simulink model "BalanceTest_MDL"  (R2016b)
settings: Solver=FixedStepAuto  StartTime=0.0  StopTime=inf  FixedStep=0.02  RelTol=1e-3
values from neighbouring files (symbols this model uses):
  alpha_comp = 0.98    [ModelSetup.m]
  K_phi = 2.42    [ModelSetup.m]
  K_u_K = 0.3    [ModelSetup.m]
  K_u_R = 0.0008    [ModelSetup.m]
  phi_max = degtorad(10)    [ModelSetup.m]
  r_S1 = 0.14    [ModelSetup.m]
  r_S2 = 0.061    [ModelSetup.m]
  Ta = 0.02    [ModelSetup.m]
undefined symbols (not defined in the file or in its folder): adc_poly, w1_poly, w2_poly, x1_poly, x2_poly, y1_poly, y2_poly
libraries: MSCubeLibrary x3, simulink x1
settings Model: SimulationMode=external  Creator=ich  LastModifiedBy=ich
settings OptimizationCC: MaxStackSize=64
settings DebuggingCC: ParameterTunabilityLossMsg=error
settings HardwareCC: ProdBitPerPointer=32  ProdBitPerSizeT=32  ProdBitPerPtrDiffT=32  ProdLargestAtomicInteger=Long  ProdLargestAtomicFloat=Double  ProdWordSize=32  ProdHWDeviceType=ARM Compatible->ARM Cortex
settings RTWCC: SystemTargetFile=ert.tlc  HardwareBoard=MSCubeBBB  TLCOptions="-aInlineSetEventsForThisBaseRateFcn=TLC_FALSE -aSuppressMultiTaskScheduler=TLC_FALSE  -aRateBasedStepFcn=0"  TemplateMakefile=ert_default_tmf  Description=Embedded Coder  GenerateReport=on  Toolchain=Linaro Toolchain v4.8  IncludeHyperlinkInReport=on  LaunchReport=on  GenerateTraceInfo=on  GenerateTraceReport=on  GenerateTraceReportSl=on  GenerateTraceReportSf=on  GenerateTraceReportEml=on
settings CodeAppCC: ForceParamTrailComments=on  IgnoreCustomStorageClasses=off  OperatorAnnotations=on  SimulinkDataObjDesc=on  SFDataObjDesc=on  MATLABFcnDesc=on  InsertBlockDesc=on  MATLABSourceComments=on

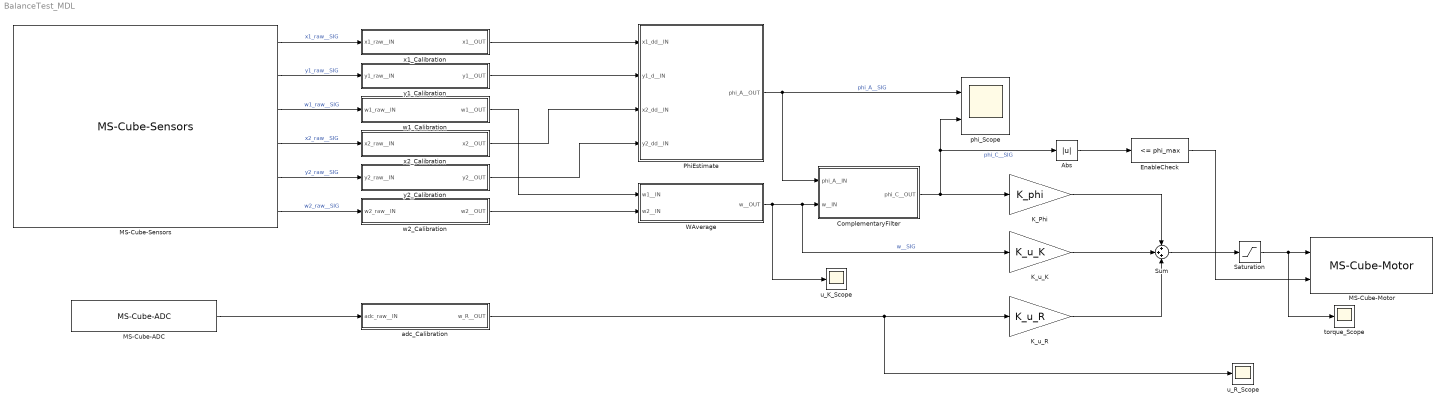
== system BalanceTest_MDL ==
  Abs : Abs
  ComplementaryFilter : Subsystem
  EnableCheck : simulink/Logic and Bit Operations/Compare To Constant  relop=<=  const=phi_max  OutDataTypeStr=boolean
  K_Phi : Gain  Gain=K_phi
  K_u_K : Gain  Gain=K_u_K
  K_u_R : Gain  Gain=K_u_R
  MS-Cube-ADC : MSCubeLibrary/MS-Cube-ADC
  MS-Cube-Motor : MSCubeLibrary/MS-Cube-Motor
  MS-Cube-Sensors : MSCubeLibrary/MS-Cube-Sensors
  PhiEstimate : Subsystem
  Saturation : Saturate  UpperLimit=0.11  LowerLimit=-0.11  OutDataTypeStr=single
  Sum : Sum  Inputs=+++  OutDataTypeStr=single
  WAverage : Subsystem
  adc_Calibration : Subsystem
  phi_Scope : Scope  NumInputPorts=2
  torque_Scope : Scope
  u_K_Scope : Scope
  u_R_Scope : Scope
  w1_Calibration : Subsystem
  w2_Calibration : Subsystem
  x1_Calibration : Subsystem
  x2_Calibration : Subsystem
  y1_Calibration : Subsystem
  y2_Calibration : Subsystem
  wires:
  MS-Cube-Sensors/1 -> x1_Calibration/1(x1_raw__IN)  "x1_raw__SIG"
  MS-Cube-Sensors/2 -> y1_Calibration/1(y1_raw__IN)  "y1_raw__SIG"
  MS-Cube-Sensors/3 -> w1_Calibration/1(w1_raw__IN)  "w1_raw__SIG"
  MS-Cube-Sensors/4 -> x2_Calibration/1(x2_raw__IN)  "x2_raw__SIG"
  MS-Cube-Sensors/5 -> y2_Calibration/1(y2_raw__IN)  "y2_raw__SIG"
  MS-Cube-Sensors/6 -> w2_Calibration/1(w2_raw__IN)  "w2_raw__SIG"
  x1_Calibration/1(x1__OUT) -> PhiEstimate/1(x1_dd__IN)
  y1_Calibration/1(y1__OUT) -> PhiEstimate/2(y1_d__IN)
  x2_Calibration/1(x2__OUT) -> PhiEstimate/3(x2_dd__IN)
  y2_Calibration/1(y2__OUT) -> PhiEstimate/4(y2_dd__IN)
  w2_Calibration/1(w2__OUT) -> WAverage/2(w2__IN)
  w1_Calibration/1(w1__OUT) -> WAverage/1(w1__IN)
  PhiEstimate/1(phi_A__OUT) -> ComplementaryFilter/1(phi_A__IN), phi_Scope/1  "phi_A__SIG"
  WAverage/1(w__OUT) -> u_K_Scope/1, K_u_K/1, ComplementaryFilter/2(w__IN)  "w__SIG"
  ComplementaryFilter/1(phi_C__OUT) -> K_Phi/1, phi_Scope/2, Abs/1  "phi_C__SIG"
  MS-Cube-ADC/1 -> adc_Calibration/1(adc_raw__IN)
  K_u_K/1 -> Sum/2
  K_Phi/1 -> Sum/1
  K_u_R/1 -> Sum/3
  adc_Calibration/1(w_R__OUT) -> u_R_Scope/1, K_u_R/1
  Sum/1 -> Saturation/1
  Abs/1 -> EnableCheck/1
  EnableCheck/1 -> MS-Cube-Motor/2
  Saturation/1 -> torque_Scope/1, MS-Cube-Motor/1

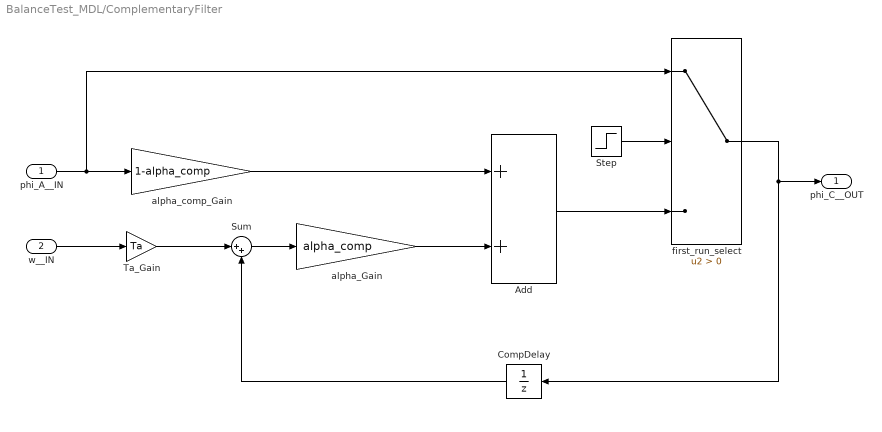
== system BalanceTest_MDL/ComplementaryFilter ==
  phi_A__IN : Inport
  w__IN : Inport  Port=2
  Add : Sum
  CompDelay : UnitDelay  SampleTime=Ta
  Step : Step  Time=Ta  Before=1  After=0  SampleTime=Ta
  Sum : Sum  Inputs=|++
  Ta_Gain : Gain  Gain=Ta
  alpha_Gain : Gain  Gain=alpha_comp
  alpha_comp_Gain : Gain  Gain=1-alpha_comp
  first_run_select : Switch  Criteria=u2 > Threshold
  phi_C__OUT : Outport
  wires:
  w__IN/1 -> Ta_Gain/1
  Ta_Gain/1 -> Sum/1
  Sum/1 -> alpha_Gain/1
  phi_A__IN/1 -> first_run_select/1, alpha_comp_Gain/1
  alpha_comp_Gain/1 -> Add/1
  alpha_Gain/1 -> Add/2
  Add/1 -> first_run_select/3
  first_run_select/1 -> CompDelay/1, phi_C__OUT/1
  CompDelay/1 -> Sum/2
  Step/1 -> first_run_select/2

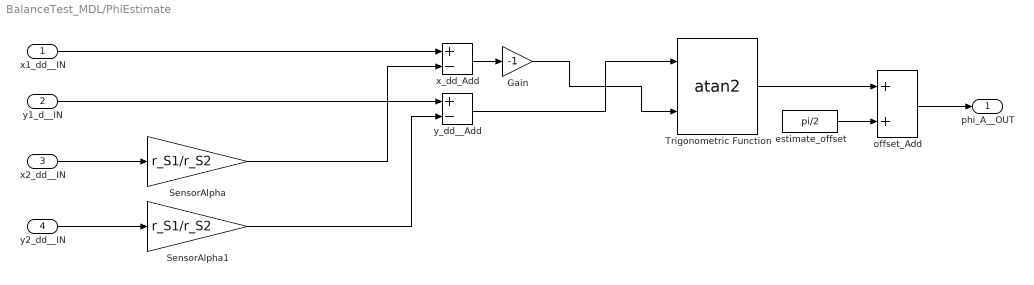
== system BalanceTest_MDL/PhiEstimate ==
  x1_dd__IN : Inport
  y1_d__IN : Inport  Port=2
  x2_dd__IN : Inport  Port=3
  y2_dd__IN : Inport  Port=4
  Gain : Gain  Gain=-1
  SensorAlpha : Gain  Gain=r_S1/r_S2
  SensorAlpha1 : Gain  Gain=r_S1/r_S2
  Trigonometric Function : Trigonometry  Operator=atan2
  estimate_offset : Constant  Value=pi/2
  offset_Add : Sum
  x_dd_Add : Sum  Inputs=+-
  y_dd__Add : Sum  Inputs=+-
  phi_A__OUT : Outport
  wires:
  x2_dd__IN/1 -> SensorAlpha/1
  y2_dd__IN/1 -> SensorAlpha1/1
  x1_dd__IN/1 -> x_dd_Add/1
  SensorAlpha/1 -> x_dd_Add/2
  y1_d__IN/1 -> y_dd__Add/1
  SensorAlpha1/1 -> y_dd__Add/2
  x_dd_Add/1 -> Gain/1
  y_dd__Add/1 -> Trigonometric Function/1
  Gain/1 -> Trigonometric Function/2
  Trigonometric Function/1 -> offset_Add/1
  estimate_offset/1 -> offset_Add/2
  offset_Add/1 -> phi_A__OUT/1

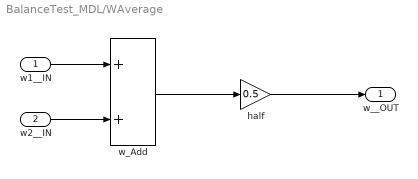
== system BalanceTest_MDL/WAverage ==
  w1__IN : Inport
  w2__IN : Inport  Port=2
  half : Gain  Gain=0.5
  w_Add : Sum
  w__OUT : Outport
  wires:
  w2__IN/1 -> w_Add/2
  w1__IN/1 -> w_Add/1
  w_Add/1 -> half/1
  half/1 -> w__OUT/1

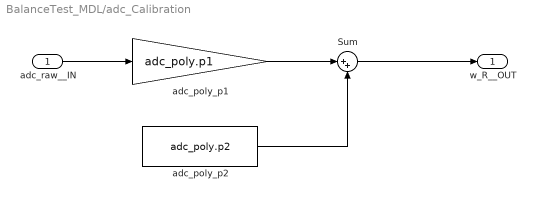
== system BalanceTest_MDL/adc_Calibration ==
  adc_raw__IN : Inport
  Sum : Sum  Inputs=|++
  adc_poly_p1 : Gain  Gain=adc_poly.p1
  adc_poly_p2 : Constant  Value=adc_poly.p2
  w_R__OUT : Outport
  wires:
  Sum/1 -> w_R__OUT/1
  adc_poly_p2/1 -> Sum/2
  adc_poly_p1/1 -> Sum/1
  adc_raw__IN/1 -> adc_poly_p1/1

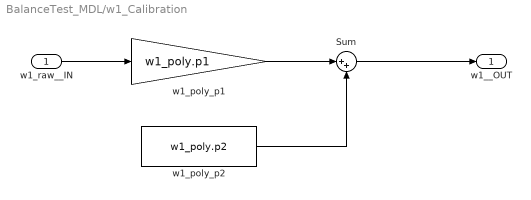
== system BalanceTest_MDL/w1_Calibration ==
  w1_raw__IN : Inport
  Sum : Sum  Inputs=|++
  w1_poly_p1 : Gain  Gain=w1_poly.p1
  w1_poly_p2 : Constant  Value=w1_poly.p2
  w1__OUT : Outport
  wires:
  Sum/1 -> w1__OUT/1
  w1_poly_p2/1 -> Sum/2
  w1_poly_p1/1 -> Sum/1
  w1_raw__IN/1 -> w1_poly_p1/1

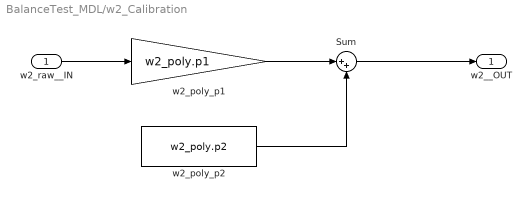
== system BalanceTest_MDL/w2_Calibration ==
  w2_raw__IN : Inport
  Sum : Sum  Inputs=|++
  w2_poly_p1 : Gain  Gain=w2_poly.p1
  w2_poly_p2 : Constant  Value=w2_poly.p2
  w2__OUT : Outport
  wires:
  w2_raw__IN/1 -> w2_poly_p1/1
  w2_poly_p1/1 -> Sum/1
  w2_poly_p2/1 -> Sum/2
  Sum/1 -> w2__OUT/1

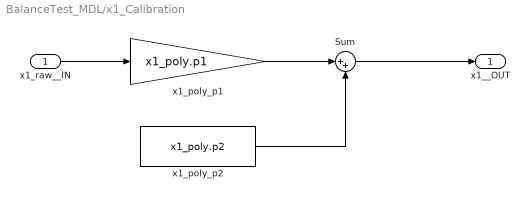
== system BalanceTest_MDL/x1_Calibration ==
  x1_raw__IN : Inport
  Sum : Sum  Inputs=|++
  x1_poly_p1 : Gain  Gain=x1_poly.p1
  x1_poly_p2 : Constant  Value=x1_poly.p2
  x1__OUT : Outport
  wires:
  Sum/1 -> x1__OUT/1
  x1_poly_p2/1 -> Sum/2
  x1_poly_p1/1 -> Sum/1
  x1_raw__IN/1 -> x1_poly_p1/1

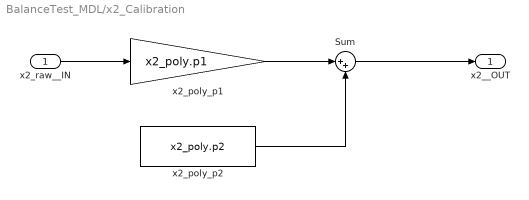
== system BalanceTest_MDL/x2_Calibration ==
  x2_raw__IN : Inport
  Sum : Sum  Inputs=|++
  x2_poly_p1 : Gain  Gain=x2_poly.p1
  x2_poly_p2 : Constant  Value=x2_poly.p2
  x2__OUT : Outport
  wires:
  x2_raw__IN/1 -> x2_poly_p1/1
  x2_poly_p1/1 -> Sum/1
  x2_poly_p2/1 -> Sum/2
  Sum/1 -> x2__OUT/1

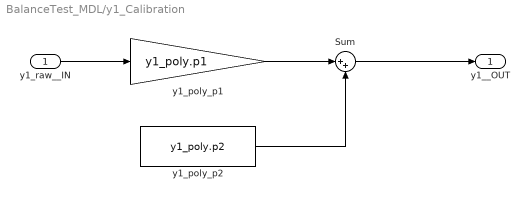
== system BalanceTest_MDL/y1_Calibration ==
  y1_raw__IN : Inport
  Sum : Sum  Inputs=|++
  y1_poly_p1 : Gain  Gain=y1_poly.p1
  y1_poly_p2 : Constant  Value=y1_poly.p2
  y1__OUT : Outport
  wires:
  y1_raw__IN/1 -> y1_poly_p1/1
  y1_poly_p1/1 -> Sum/1
  y1_poly_p2/1 -> Sum/2
  Sum/1 -> y1__OUT/1

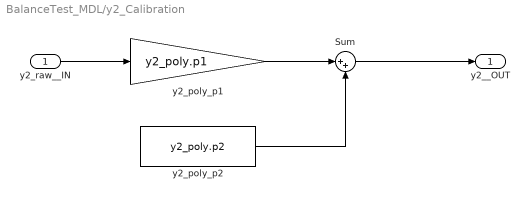
== system BalanceTest_MDL/y2_Calibration ==
  y2_raw__IN : Inport
  Sum : Sum  Inputs=|++
  y2_poly_p1 : Gain  Gain=y2_poly.p1
  y2_poly_p2 : Constant  Value=y2_poly.p2
  y2__OUT : Outport
  wires:
  Sum/1 -> y2__OUT/1
  y2_poly_p2/1 -> Sum/2
  y2_poly_p1/1 -> Sum/1
  y2_raw__IN/1 -> y2_poly_p1/1
